simulink model "DriverInLoopGamingEngine"  (R2020b)
settings: Solver=ode3  StartTime=0.0  StopTime=inf  FixedStep=1e-3  RelTol=1e-3
StartFcn:
  | tg.load('DriverInLoopSpeedgoat');
  | tg.start;
StopFcn:
  | tg.stop;
model workspace (MAT data in the model file):
  A_mu = 10
  AxlIxx = 62.3745166667
  AxlM = 160
  B_reff = 8.386
  Cps = 2
  Cz = 5565.2246438
  CzWhlAxl = 11490.971257
  DCT_Param : object (value not decoded)
  DLC_XEnd = 236.9
  DLC_XStart = 175.9
  D_reff = 0.25826
  Downshift_Speeds = [9.5625 12.9375 16.3125 19.6875 23.0625 26.4375 29.8125 33.1875 36.5625 39.9375 43.3125 46.6875 ... (28 elements, 4x7)]
  F0z = [2886 2907]
  F0zWhlAxl = 2907
  Hmax = 0.25
  Kz = 52451.0065793
  KzWhlAxl = 138031.612078
  NCyl = 6
  Pedal_Positions = [0.1 0.4 0.5 0.9]
  Pstd = 101325
  Rair = 287
  SUS : object (value not decoded)
  Sig : Simulink.Signal (value not decoded)
  Sig1 : Simulink.Signal (value not decoded)
  Sig2 : Simulink.Signal (value not decoded)
  Sig3 : Simulink.Signal (value not decoded)
  Sig4 : Simulink.Signal (value not decoded)
  Sig5 : Simulink.Signal (value not decoded)
  Sig6 : Simulink.Signal (value not decoded)
  Sig7 : Simulink.Signal (value not decoded)
  Sig8 : Simulink.Signal (value not decoded)
  Trans : object (value not decoded)
  Tstd = 293.15
  Upshift_Speeds = [12.9375 16.3125 19.6875 33 26.4375 29.8125 33.1875 52.5 39.9375 43.3125 46.6875 77.25 ... (28 elements, 4x7)]
  VEH : object (value not decoded)
  V_o = 16.7
  V_xlow = 1
  Vd = 0.00346
  WH : Mass (value not decoded)
  Y0 = 3.2153
  a = 1.4
  alpha_max = 1.5
  alpha_min = -1.5
  b = 1.8
  c_zo = 209651
  dt3D = 0.05
  epsilon = 0.1
  f_air = [0 0 0 0 0 0 0 0 0 0 0 0 ... (256 elements, 16x16)]
  f_co = [0 0 0 0 0 0 0 0 0 0 0 0 ... (256 elements, 16x16)]
  f_co2 = [0 0 0 0 0 0 0 0 0 0 0 0 ... (256 elements, 16x16)]
  f_eff = [352.135682859 352.135682859 320.724378192 303.655312657 295.930136708 291.240087194 291.240271258 291.240312459 291.240275452 291.240198499 291.240100781 291.240018769 ... (256 elements, 16x16)]
  f_fuel = [0 0 0 0 0 0 0 0 0 0 0 0 ... (256 elements, 16x16)]
  f_hc = [0 0 0 0 0 0 0 0 0 0 0 0 ... (256 elements, 16x16)]
  f_nox = [0 0 0 0 0 0 0 0 0 0 0 0 ... (256 elements, 16x16)]
  f_pm = [0 0 0 0 0 0 0 0 0 0 0 0 ... (256 elements, 16x16)]
  f_susp_axl_bp = [1 2]
  f_susp_dz_bp = [-0.325022776267 -0.315022776267 -0.305022776267 -0.205022776267 -0.105022776267 -0.00502277626717 0.0949772237328 0.194977223733 0.204977223733 0.214977223733]
  f_susp_dzdot_bp = [-3 -0.3 -0.2 -0.1 0 0.1 0.2 0.3 3]
  f_susp_fmz = [-144070.391448 -93629.24037 -75929.1118915 -20630.5828179 -15385.48216 -10140.3815021 -4895.28084414 349.819813785 -31916.3973792 18437.6709544 -83996.1993354 -33555.0482577 ... (43920 elements, 10x9x61x2x4)]
  f_susp_geom = [0 0 0 0 0 0 0 0 0 0 0 0 ... (3660 elements, 10x61x2x3)]
  f_susp_strgdelta_bp = [-0.523598775598 -0.506145483078 -0.488692190558 -0.471238898038 -0.453785605519 -0.436332312999 -0.418879020479 -0.401425727959 -0.383972435439 -0.366519142919 -0.349065850399 -0.331612557879 ... (61 elements, 1x61)]
  f_tbrake = [0 76.8593923996 105.140482948 131.533638111 157.926793274 176.658631717 176.65727296 176.656856686 176.656879077 176.657093756 176.657404516 176.65772406 ... (256 elements, 16x16)]
  f_tbrake_n_bpt = [0 649.519052838 912.419621844 1175.32019085 1438.22075986 1701.12132886 1964.02189787 2226.92246687 2489.82303588 2752.72360489 3015.62417389 3278.5247429 ... (16 elements, 1x16)]
  f_tbrake_t_bpt = [0 34.6410161514 61.0341713143 87.4273264773 113.82048164 140.213636803 166.606791966 192.999947129 219.393102292 245.786257455 272.179412618 298.572567781 ... (16 elements, 1x16)]
  f_texh = [766.752464599 766.752464599 786.17542386 801.679939032 884.591982581 910.574397722 910.571871054 910.570774534 910.570601632 910.570821151 910.571247242 910.571639815 ... (256 elements, 16x16)]
  f_twc_eff_co = [0.17 0.25 0.45 0.99 0.99 0.99 0.99]
  f_twc_eff_hc = [0.21 0.375 0.75 0.98 0.98 0.98 0.98]
  f_twc_eff_lam = [0.909090909 0.944055944 0.979020979 1 1.013986014 1.048951049 1.083916084]
  f_twc_eff_nox = [0.98 0.98 0.98 0.97 0.05 0.02 0]
  h = 0.134
  numWheel = 4
  path : object (value not decoded)
  pio = 220000
  q_Fcx = 0
  q_Fz2 = 15.4
  q_Fzy = 0
  q_reo = 0.9974
  q_sx1 = -0.007764
  q_sx10 = 0.2824
  q_sx11 = 5.349
  q_sx12 = 0
  q_sx13 = 0
  q_sx14 = 0
  q_sx2 = 1.1915
  q_sx3 = 0.013948
  q_sx4 = 4.912
  q_sx5 = 1.02
  q_sx6 = 22.83
  q_sx7 = 0.7104
  q_sx8 = -0.023393
  q_sx9 = 0.6581
  q_sy1 = 0.00702
  q_sy2 = 0
  q_sy3 = 0.001515
  q_sy4 = 8.514e-05
  q_sy5 = 0
  q_sy6 = 0
  q_sy7 = 0.9008
  q_sy8 = -0.4089
  q_v1 = 0.0007742
  q_v2 = 0.04667
  r_Bx1 = 12.531
  r_Bx2 = 9.532
  r_Bx3 = 0
  r_By1 = 10.615
  r_By2 = 7.705
  r_By3 = 3.433e-06
  r_By4 = 0
  r_Cx1 = 1.019
  r_Cy1 = 1.0585
  r_Ex1 = -0.4487
  r_Ex2 = -0.4726
  r_Ey1 = 0.3132
  r_Ey2 = 7.63e-06
  r_Hx1 = 0.0002374
  r_Hy1 = 0.011646
  r_Hy2 = 7.63e-06
  r_Vy1 = 0.05654
  r_Vy2 = 7.63e-06
  r_Vy3 = 0
  r_Vy4 = 99.9
  r_Vy5 = 2
  r_Vy6 = 15.814
  r_o = 0.3135
  vehWidth = 2
  w = 1
  xdot_ref = 13.4112
symbols that are objects in the model workspace (value not decoded): VEH
libraries: slrealtimeutilitieslib x3, slrealtimeiplib x3, sim3dlib x2, sim3dautolib x1, dspfdesign x1, vrlib x1, simulink x1
(part 2 of 2)

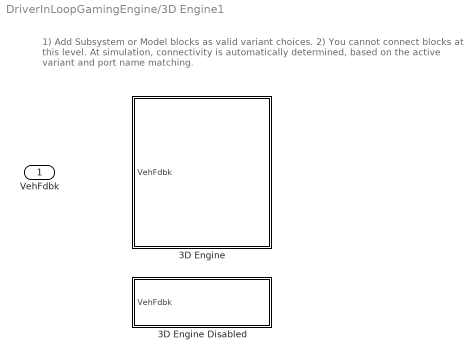
== system DriverInLoopGamingEngine/3D Engine1 ==
  note: 1) Add Subsystem or Model blocks as valid variant choices.
      | 2) You cannot connect blocks at this level. At simulation, connectivity is automatically
      | determined, based on the active variant and port name matching.
  VehFdbk : Inport
  3D Engine : Subsystem  VariantControl=1
  3D Engine Disabled : Subsystem  VariantControl=0

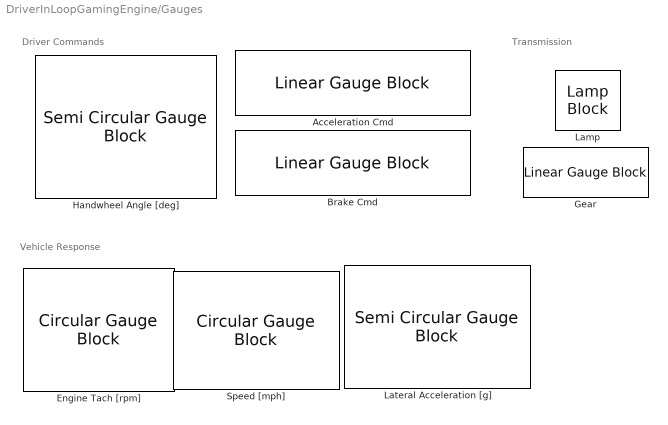
== system DriverInLoopGamingEngine/Gauges ==
  note: Vehicle Response
  note: Driver Commands
  note: Transmission
  Acceleration Cmd : LinearGaugeBlock  ScaleMax=1
  Brake Cmd : LinearGaugeBlock  ScaleMax=1
  Engine Tach [rpm] : CircularGaugeBlock  ScaleMax=8000  TickInterval=1000
  Gear : LinearGaugeBlock  ScaleMin=-1  ScaleMax=5  TickInterval=1
  Handwheel Angle [deg] : SemiCircularGaugeBlock  ScaleMin=-450  ScaleMax=450  TickInterval=90
  Lamp : LampBlock
  Lateral Acceleration [g] : SemiCircularGaugeBlock  ScaleMin=-1  ScaleMax=1  TickInterval=0.5
  Speed [mph] : CircularGaugeBlock

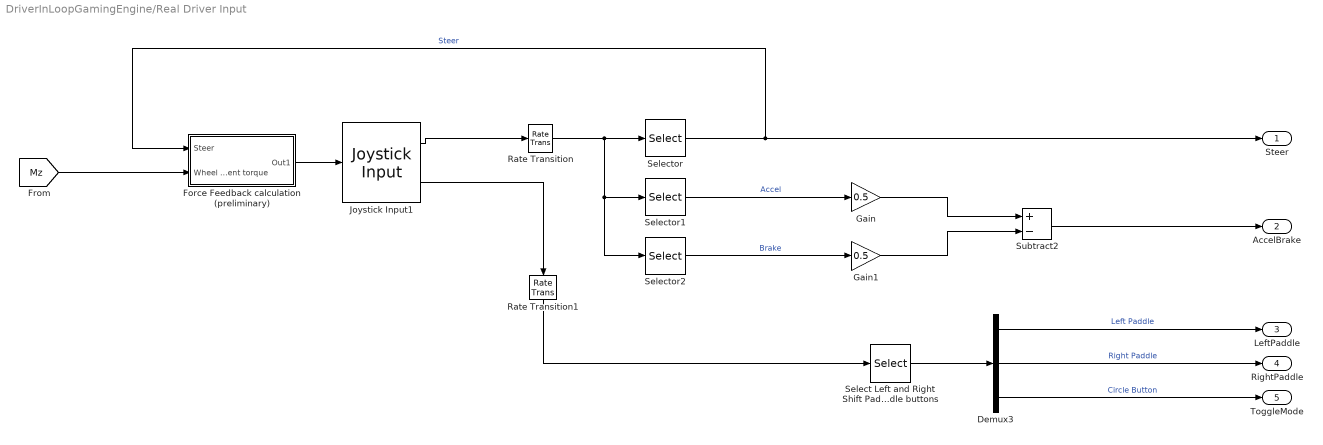
== system DriverInLoopGamingEngine/Real Driver Input ==
  Demux3 : Demux  Outputs=3
  Force Feedback calculation (preliminary) : Subsystem
  Gain : Gain  Gain=0.5
  Gain1 : Gain  Gain=0.5
  Joystick Input1 : vrlib/Joystick Input  joyid=1  adjustports=on  forcefeed=on
  Rate Transition : RateTransition  Deterministic=off
  Rate Transition1 : RateTransition  Deterministic=off
  Select Left and Right Shift Paddle buttons : Selector  InputPortWidth=25  IndexOptions=Index vector (dialog)  Indices=[6 5 3]  OutputSizes=1
  Selector : Selector  InputPortWidth=4  IndexOptions=Index vector (dialog)  Indices=1  OutputSizes=1
  Selector1 : Selector  InputPortWidth=4  IndexOptions=Index vector (dialog)  Indices=2  OutputSizes=1
  Selector2 : Selector  InputPortWidth=4  IndexOptions=Index vector (dialog)  Indices=3  OutputSizes=1
  Subtract2 : Sum  Inputs=+-
  Steer : Outport  VectorParamsAs1DForOutWhenUnconnected=off
  AccelBrake : Outport  Port=2  VectorParamsAs1DForOutWhenUnconnected=off
  LeftPaddle : Outport  Port=3  VectorParamsAs1DForOutWhenUnconnected=off
  RightPaddle : Outport  Port=4  VectorParamsAs1DForOutWhenUnconnected=off
  ToggleMode : Outport  Port=5  VectorParamsAs1DForOutWhenUnconnected=off
  wires:
  Joystick Input1/1 -> Rate Transition/1
  Rate Transition1/1 -> Select Left and Right Shift Paddle buttons/1
  Demux3/2 -> RightPaddle/1  "Right Paddle"
  Demux3/1 -> LeftPaddle/1  "Left Paddle"
  Select Left and Right Shift Paddle buttons/1 -> Demux3/1
  Rate Transition/1 -> Selector2/1, Selector1/1, Selector/1
  Joystick Input1/2 -> Rate Transition1/1
  Selector1/1 -> Gain/1  "Accel"
  Selector2/1 -> Gain1/1  "Brake"
  Gain/1 -> Subtract2/1
  Gain1/1 -> Subtract2/2
  Subtract2/1 -> AccelBrake/1
  Demux3/3 -> ToggleMode/1  "Circle Button"
  Selector/1 -> Steer/1, Force Feedback calculation (preliminary)/1(Steer)  "Steer"
  [Mz] -> Force Feedback calculation (preliminary)/2(Wheel alignment torque)
  Force Feedback calculation (preliminary)/1(Out1) -> Joystick Input1/1

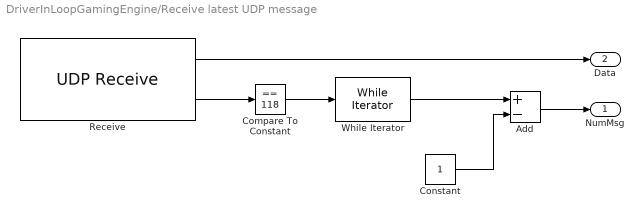
== system DriverInLoopGamingEngine/Receive latest UDP message ==
  Add : Sum  Inputs=+-
  Compare To Constant : simulink/Logic and Bit Operations/Compare To Constant  relop===  const=118  OutDataTypeStr=boolean
  Constant : Constant  OutDataTypeStr=Inherit: Inherit via back propagation  SampleTime=-1
  Receive : slrealtimeiplib/UDP Receive  useHostTargetConn=off  ipAddress=192.168.7.2  localPort=25001  rcvWidth=118  rcvFmAny=off  fmAddress=192.168.7.1  rcvMulticast=off  multicastAddress=[]  sampleTime=-1
      settings: SourceProductBaseCode=XP
  While Iterator : WhileIterator  MaxIters=10  WhileBlockType=do-while  ShowIterationPort=on
  NumMsg : Outport
  Data : Outport  Port=2
  wires:
  Receive/2 -> Compare To Constant/1
  Compare To Constant/1 -> While Iterator/1
  While Iterator/1 -> Add/1
  Constant/1 -> Add/2
  Receive/1 -> Data/1
  Add/1 -> NumMsg/1

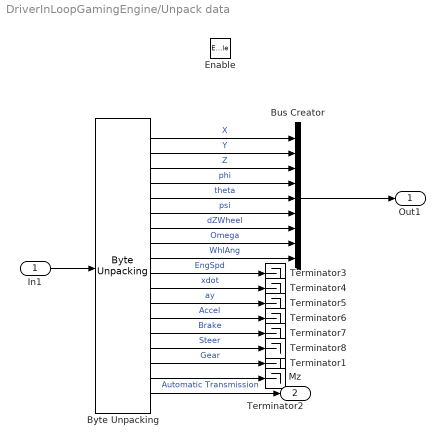
== system DriverInLoopGamingEngine/Unpack data ==
  In1 : Inport
  Enable : EnablePort
  Bus Creator : BusCreator  Inputs=9
  "Byte Unpacking " : slrealtimeutilitieslib/Byte Unpacking  MaskUnpackedDataTypes={'single','single','single','single','single','single','single','double','single','single','single','single','single','single','single','int8','int8','single'}  MaskUnpackedDataSizes={[1],[1],[1],[1],[1],[1],[4],[4],[4],[1],[1],[1],[1],[1],[1],[1],[1],[1]}  MaskAlignment=1
      settings: SourceProductBaseCode=XP
  Terminator{1..8} (8 alike) : Terminator
  Out1 : Outport
  Mz : Outport  Port=2
  wires:
  "Byte Unpacking "/8 -> Bus Creator/8  "Omega"
  "Byte Unpacking "/14 -> Terminator7/1  "Brake"
  "Byte Unpacking "/7 -> Bus Creator/7  "dZWheel"
  "Byte Unpacking "/4 -> Bus Creator/4  "phi"
  "Byte Unpacking "/15 -> Terminator8/1  "Steer"
  "Byte Unpacking "/9 -> Bus Creator/9  "WhlAng"
  "Byte Unpacking "/13 -> Terminator6/1  "Accel"
  "Byte Unpacking "/2 -> Bus Creator/2  "Y"
  "Byte Unpacking "/10 -> Terminator3/1  "EngSpd"
  In1/1 -> "Byte Unpacking "/1
  "Byte Unpacking "/3 -> Bus Creator/3  "Z"
  "Byte Unpacking "/12 -> Terminator5/1  "ay"
  "Byte Unpacking "/11 -> Terminator4/1  "xdot"
  "Byte Unpacking "/1 -> Bus Creator/1  "X"
  "Byte Unpacking "/6 -> Bus Creator/6  "psi"
  "Byte Unpacking "/5 -> Bus Creator/5  "theta"
  Bus Creator/1 -> Out1/1
  "Byte Unpacking "/16 -> Terminator1/1  "Gear"
  "Byte Unpacking "/17 -> Terminator2/1  "Automatic Transmission"
  "Byte Unpacking "/18 -> Mz/1

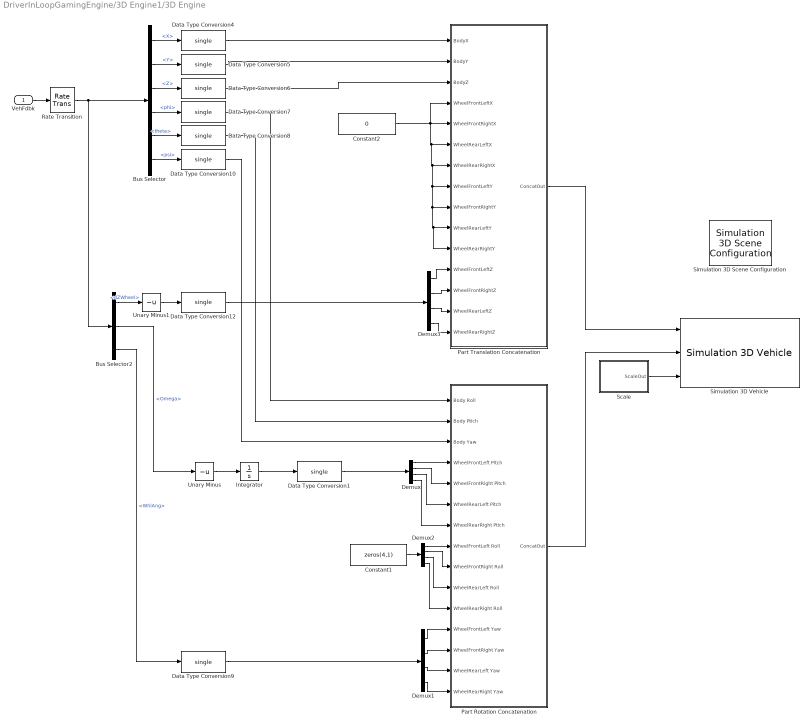
== system DriverInLoopGamingEngine/3D Engine1/3D Engine ==
  VehFdbk : Inport
  Bus Selector : BusSelector  OutputSignals=X,Y,Z,phi,theta,psi
  Bus Selector2 : BusSelector  OutputSignals=dZWheel,Omega,WhlAng
  Constant1 : Constant  Value=zeros(4,1)  OutDataTypeStr=single
  Constant2 : Constant  Value=0  OutDataTypeStr=single
  Data Type Conversion{1,4..10,12} (9 alike) : DataTypeConversion  OutDataTypeStr=single
  Demux{,1..3} (4 alike) : Demux
  Integrator : Integrator  WrapState=on  WrappedStateUpperValue=2*pi  WrappedStateLowerValue=0  ZeroCross=off
  Part Rotation Concatenation : Subsystem
  Part Translation Concatenation : Subsystem
  Rate Transition : RateTransition  Deterministic=off  OutPortSampleTime=dt3D
  Scale : Subsystem
  Simulation 3D Scene Configuration : sim3dlib/Simulation 3D Scene Configuration  Priority=0  ProjectFormat=Default Scenes  SceneDesc=Virtual Mcity  ProjectName=VehicleSimulation.exe  ScenePath=/Game/Maps/HwStrght  vehTagList={'Scene Origin';'SimulinkVehicle1'}  vehTag=SimulinkVehicle1  OpVisEn=off  Ts=dt3D  EnableWindow=on  sensorTag=MainCamera2  sensorId=2  sensorName=MainCamera2  mountLoc=Origin  offsetFlag=off  tmountOffset=[0, 0, 0]  rmountOffset=[0, 0, 0]  HorizontalResolution=1280  VerticalResolution=720  HorizontalFOV=60  mountPoint=[0 0 0]  mountOrientation=[0 0 0]  aMode=aMode  ID=2
      settings: SourceProductBaseCode=DR,UV,VE
  Simulation 3D Vehicle : sim3dautolib/Simulation 3D Vehicle  Priority=-1  PassVehMesh=Muscle car  VehColor=Red  ActorName=SimulinkVehicle1  Translation=[VEH.InitialLongPosition VEH.InitialLatPosition -VEH.InitialVertPosition; 0 0 0; 0 0 0; 0 0 0; 0 0 0]  Rotation=[VEH.InitialRollAngle VEH.InitialPitchAngle VEH.InitialYawAngle; 0 0 0; 0 0 0; 0 0 0; 0 0 0]  Scale=ones( 5, 3 )  SampleTime=dt3D  ActorType=SimulinkVehicle  ID=1  aMode=2  ActorTag=SimulinkVehicle1
      settings: SourceProductBaseCode=DR,UV,VE
  Unary Minus : UnaryMinus
  Unary Minus1 : UnaryMinus
  wires:
  Unary Minus/1 -> Integrator/1
  Bus Selector2/1 -> Unary Minus1/1  "<dZWheel>"
  Rate Transition/1 -> Bus Selector/1, Bus Selector2/1
  Scale/1(ScaleOut) -> Simulation 3D Vehicle/3
  Demux/4 -> Part Rotation Concatenation/7(WheelRearRight Ptich)
  Demux/3 -> Part Rotation Concatenation/6(WheelRearLeft Pitch)
  Demux/2 -> Part Rotation Concatenation/5(WheelFrontRight Pitch)
  Demux/1 -> Part Rotation Concatenation/4(WheelFrontLeft Pitch)
  Constant1/1 -> Demux2/1
  Bus Selector/4 -> Data Type Conversion7/1  "<phi>"
  Part Rotation Concatenation/1(ConcatOut) -> Simulation 3D Vehicle/2
  Part Translation Concatenation/1(ConcatOut) -> Simulation 3D Vehicle/1
  Data Type Conversion12/1 -> Demux3/1
  Demux3/4 -> Part Translation Concatenation/15(WheelRearRightZ)
  Demux3/3 -> Part Translation Concatenation/14(WheelRearLeftZ)
  Demux3/1 -> Part Translation Concatenation/12(WheelFrontLeftZ)
  Demux3/2 -> Part Translation Concatenation/13(WheelFrontRightZ)
  VehFdbk/1 -> Rate Transition/1
  Data Type Conversion6/1 -> Part Translation Concatenation/3(BodyZ)
  Demux1/4 -> Part Rotation Concatenation/15(WheelRearRight Yaw)
  Demux1/3 -> Part Rotation Concatenation/14(WheelRearLeft Yaw)
  Demux2/1 -> Part Rotation Concatenation/8(WheelFrontLeft Roll)
  Demux2/2 -> Part Rotation Concatenation/9(WheelFrontRight Roll)
  Demux2/3 -> Part Rotation Concatenation/10(WheelRearLeft Roll)
  Demux2/4 -> Part Rotation Concatenation/11(WheelRearRight Roll)
  Bus Selector2/3 -> Data Type Conversion9/1  "<WhlAng>"
  Bus Selector2/2 -> Unary Minus/1  "<Omega>"
  Data Type Conversion9/1 -> Demux1/1
  Demux1/1 -> Part Rotation Concatenation/12(WheelFrontLeft Yaw)
  Demux1/2 -> Part Rotation Concatenation/13(WheelFrontRight Yaw)
  Integrator/1 -> Data Type Conversion1/1
  Data Type Conversion1/1 -> Demux/1
  Data Type Conversion8/1 -> Part Rotation Concatenation/2(Body Ptich)
  Data Type Conversion5/1 -> Part Translation Concatenation/2(BodyY)
  Data Type Conversion10/1 -> Part Rotation Concatenation/3(Body Yaw)
  Constant2/1 -> Part Translation Concatenation/5(WheelFrontRightX), Part Translation Concatenation/6(WheelRearLeftX), Part Translation Concatenation/7(WheelRearRightX), Part Translation Concatenation/8(WheelFrontLeftY), Part Translation Concatenation/9(WheelFrontRightY), Part Translation Concatenation/10(WheelRearLeftY), Part Translation Concatenation/11(WheelRearRightY), Part Translation Concatenation/4(WheelFrontLeftX)
  Data Type Conversion4/1 -> Part Translation Concatenation/1(BodyX)
  Data Type Conversion7/1 -> Part Rotation Concatenation/1(Body Roll)
  Bus Selector/1 -> Data Type Conversion4/1  "<X>"
  Bus Selector/2 -> Data Type Conversion5/1  "<Y>"
  Bus Selector/3 -> Data Type Conversion6/1  "<Z>"
  Bus Selector/6 -> Data Type Conversion10/1  "<psi>"
  Bus Selector/5 -> Data Type Conversion8/1  "<theta>"
  Unary Minus1/1 -> Data Type Conversion12/1

== system DriverInLoopGamingEngine/3D Engine1/3D Engine Disabled ==
  VehFdbk : Inport
  Terminator : Terminator
  wires:
  VehFdbk/1 -> Terminator/1

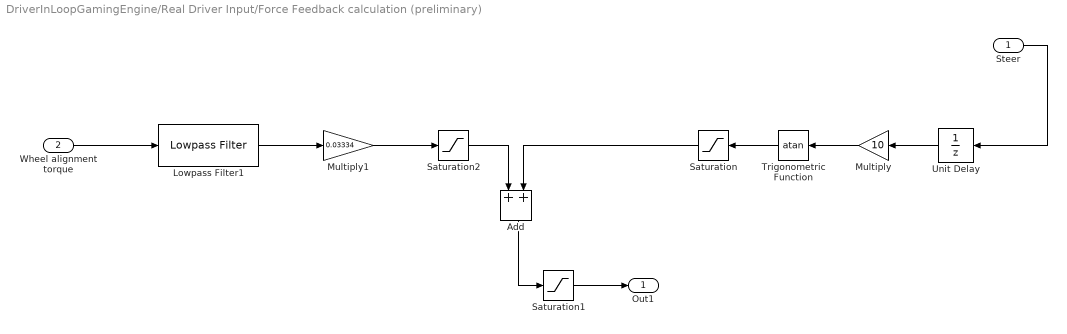
== system DriverInLoopGamingEngine/Real Driver Input/Force Feedback calculation (preliminary) ==
  Steer : Inport
  Wheel alignment torque : Inport  Port=2
  Add : Sum
  Lowpass Filter1 : dspfdesign/Lowpass Filter  FilterType=FIR  DesignForMinimumOrder=on  FilterOrder=50  PassbandFrequency=1  StopbandFrequency=40  PassbandRipple=0.1  StopbandAttenuation=80  InheritSampleRate=off  SampleRate=1000  SimulateUsing=Interpreted execution  roundingMode=Floor  coeffsDataTypeStr=fixdt(1,16)
  Multiply : Gain  Gain=10
  Multiply1 : Gain  Gain=0.03334
  Saturation : Saturate  UpperLimit=0.6  LowerLimit=-0.6
  Saturation1 : Saturate  UpperLimit=1  LowerLimit=-1
  Saturation2 : Saturate  UpperLimit=0.6  LowerLimit=-0.6
  Trigonometric Function : Trigonometry  Operator=atan  OutputSignalType=real
  Unit Delay : UnitDelay  SampleTime=-1  HasFrameUpgradeWarning=on
  Out1 : Outport
  wires:
  Multiply/1 -> Trigonometric Function/1
  Unit Delay/1 -> Multiply/1
  Saturation1/1 -> Out1/1
  Saturation/1 -> Add/2
  Multiply1/1 -> Saturation2/1
  Trigonometric Function/1 -> Saturation/1
  Add/1 -> Saturation1/1
  Lowpass Filter1/1 -> Multiply1/1
  Saturation2/1 -> Add/1
  Steer/1 -> Unit Delay/1
  Wheel alignment torque/1 -> Lowpass Filter1/1

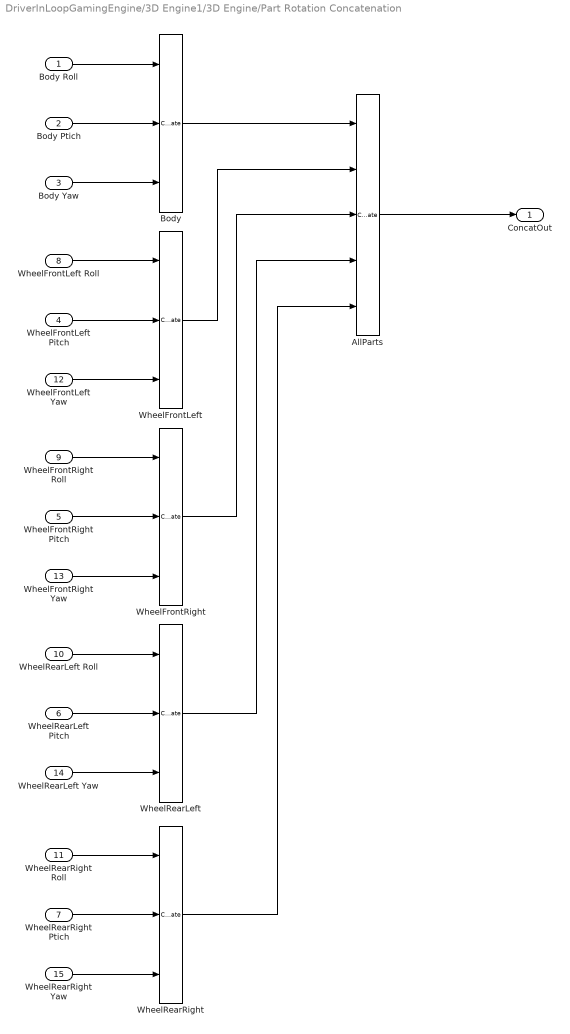
== system DriverInLoopGamingEngine/3D Engine1/3D Engine/Part Rotation Concatenation ==
  Body Roll : Inport
  Body Ptich : Inport  Port=2
  Body Yaw : Inport  Port=3
  WheelFrontLeft Pitch : Inport  Port=4
  WheelFrontRight Pitch : Inport  Port=5
  WheelRearLeft Pitch : Inport  Port=6
  WheelRearRight Ptich : Inport  Port=7
  WheelFrontLeft Roll : Inport  Port=8
  WheelFrontRight Roll : Inport  Port=9
  WheelRearLeft Roll : Inport  Port=10
  WheelRearRight Roll : Inport  Port=11
  WheelFrontLeft Yaw : Inport  Port=12
  WheelFrontRight Yaw : Inport  Port=13
  WheelRearLeft Yaw : Inport  Port=14
  WheelRearRight Yaw : Inport  Port=15
  AllParts : Concatenate  NumInputs=5  Mode=Multidimensional array
  Body : Concatenate  NumInputs=3  Mode=Multidimensional array  ConcatenateDimension=2
  WheelFrontLeft : Concatenate  NumInputs=3  Mode=Multidimensional array  ConcatenateDimension=2
  WheelFrontRight : Concatenate  NumInputs=3  Mode=Multidimensional array  ConcatenateDimension=2
  WheelRearLeft : Concatenate  NumInputs=3  Mode=Multidimensional array  ConcatenateDimension=2
  WheelRearRight : Concatenate  NumInputs=3  Mode=Multidimensional array  ConcatenateDimension=2
  ConcatOut : Outport  VectorParamsAs1DForOutWhenUnconnected=off
  wires:
  Body Yaw/1 -> Body/3
  WheelFrontLeft Yaw/1 -> WheelFrontLeft/3
  WheelFrontLeft/1 -> AllParts/2
  Body/1 -> AllParts/1
  WheelRearLeft/1 -> AllParts/4
  WheelFrontRight/1 -> AllParts/3
  WheelRearRight Yaw/1 -> WheelRearRight/3
  WheelRearLeft Yaw/1 -> WheelRearLeft/3
  AllParts/1 -> ConcatOut/1
  WheelRearRight/1 -> AllParts/5
  WheelFrontRight Yaw/1 -> WheelFrontRight/3
  Body Roll/1 -> Body/1
  Body Ptich/1 -> Body/2
  WheelFrontLeft Pitch/1 -> WheelFrontLeft/2
  WheelFrontLeft Roll/1 -> WheelFrontLeft/1
  WheelFrontRight Roll/1 -> WheelFrontRight/1
  WheelFrontRight Pitch/1 -> WheelFrontRight/2
  WheelRearLeft Roll/1 -> WheelRearLeft/1
  WheelRearLeft Pitch/1 -> WheelRearLeft/2
  WheelRearRight Roll/1 -> WheelRearRight/1
  WheelRearRight Ptich/1 -> WheelRearRight/2

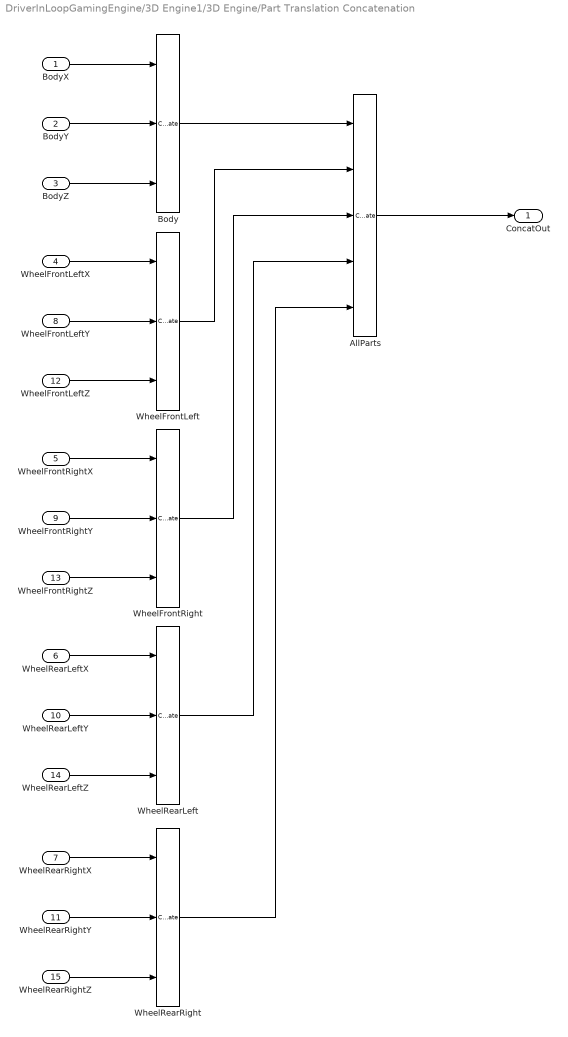
== system DriverInLoopGamingEngine/3D Engine1/3D Engine/Part Translation Concatenation ==
  BodyX : Inport
  BodyY : Inport  Port=2
  BodyZ : Inport  Port=3
  WheelFrontLeftX : Inport  Port=4
  WheelFrontRightX : Inport  Port=5
  WheelRearLeftX : Inport  Port=6
  WheelRearRightX : Inport  Port=7
  WheelFrontLeftY : Inport  Port=8
  WheelFrontRightY : Inport  Port=9
  WheelRearLeftY : Inport  Port=10
  WheelRearRightY : Inport  Port=11
  WheelFrontLeftZ : Inport  Port=12
  WheelFrontRightZ : Inport  Port=13
  WheelRearLeftZ : Inport  Port=14
  WheelRearRightZ : Inport  Port=15
  AllParts : Concatenate  NumInputs=5  Mode=Multidimensional array
  Body : Concatenate  NumInputs=3  Mode=Multidimensional array  ConcatenateDimension=2
  WheelFrontLeft : Concatenate  NumInputs=3  Mode=Multidimensional array  ConcatenateDimension=2
  WheelFrontRight : Concatenate  NumInputs=3  Mode=Multidimensional array  ConcatenateDimension=2
  WheelRearLeft : Concatenate  NumInputs=3  Mode=Multidimensional array  ConcatenateDimension=2
  WheelRearRight : Concatenate  NumInputs=3  Mode=Multidimensional array  ConcatenateDimension=2
  ConcatOut : Outport  VectorParamsAs1DForOutWhenUnconnected=off
  wires:
  BodyX/1 -> Body/1
  BodyZ/1 -> Body/3
  WheelFrontLeftX/1 -> WheelFrontLeft/1
  WheelFrontLeftZ/1 -> WheelFrontLeft/3
  WheelFrontLeftY/1 -> WheelFrontLeft/2
  BodyY/1 -> Body/2
  WheelFrontLeft/1 -> AllParts/2
  WheelRearRightX/1 -> WheelRearRight/1
  Body/1 -> AllParts/1
  WheelRearLeft/1 -> AllParts/4
  WheelFrontRight/1 -> AllParts/3
  WheelRearRightZ/1 -> WheelRearRight/3
  WheelFrontRightY/1 -> WheelFrontRight/2
  WheelFrontRightX/1 -> WheelFrontRight/1
  WheelRearRightY/1 -> WheelRearRight/2
  WheelRearLeftZ/1 -> WheelRearLeft/3
  AllParts/1 -> ConcatOut/1
  WheelRearLeftY/1 -> WheelRearLeft/2
  WheelRearRight/1 -> AllParts/5
  WheelRearLeftX/1 -> WheelRearLeft/1
  WheelFrontRightZ/1 -> WheelFrontRight/3

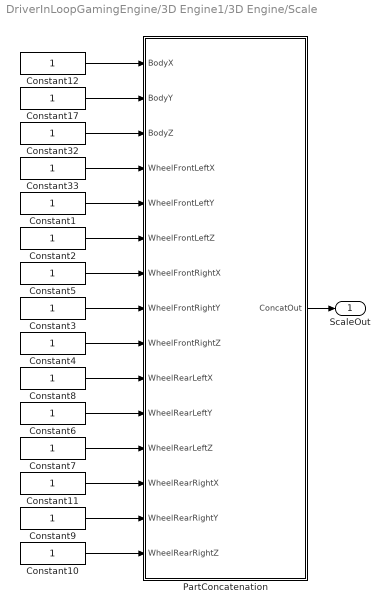
== system DriverInLoopGamingEngine/3D Engine1/3D Engine/Scale ==
  Constant{1..12,17,32..33} (15 alike) : Constant  OutDataTypeStr=single
  PartConcatenation : Subsystem
  ScaleOut : Outport  VectorParamsAs1DForOutWhenUnconnected=off
  wires:
  Constant10/1 -> PartConcatenation/15(WheelRearRightZ)
  Constant9/1 -> PartConcatenation/14(WheelRearRightY)
  Constant11/1 -> PartConcatenation/13(WheelRearRightX)
  Constant7/1 -> PartConcatenation/12(WheelRearLeftZ)
  Constant6/1 -> PartConcatenation/11(WheelRearLeftY)
  Constant8/1 -> PartConcatenation/10(WheelRearLeftX)
  Constant4/1 -> PartConcatenation/9(WheelFrontRightZ)
  Constant3/1 -> PartConcatenation/8(WheelFrontRightY)
  Constant5/1 -> PartConcatenation/7(WheelFrontRightX)
  Constant2/1 -> PartConcatenation/6(WheelFrontLeftZ)
  Constant1/1 -> PartConcatenation/5(WheelFrontLeftY)
  Constant33/1 -> PartConcatenation/4(WheelFrontLeftX)
  Constant32/1 -> PartConcatenation/3(BodyZ)
  Constant17/1 -> PartConcatenation/2(BodyY)
  Constant12/1 -> PartConcatenation/1(BodyX)
  PartConcatenation/1(ConcatOut) -> ScaleOut/1

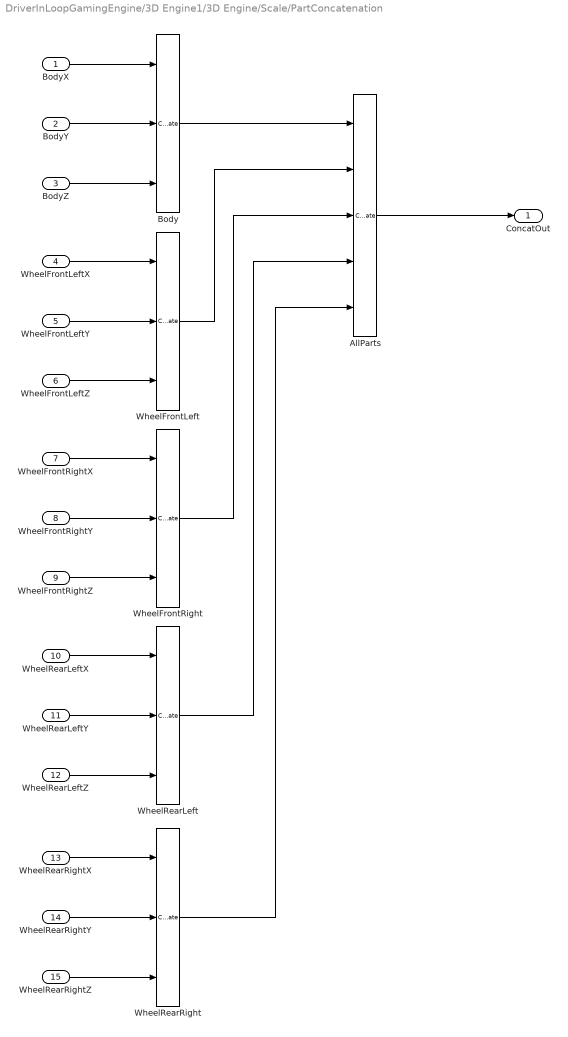
== system DriverInLoopGamingEngine/3D Engine1/3D Engine/Scale/PartConcatenation ==
  BodyX : Inport
  BodyY : Inport  Port=2
  BodyZ : Inport  Port=3
  WheelFrontLeftX : Inport  Port=4
  WheelFrontLeftY : Inport  Port=5
  WheelFrontLeftZ : Inport  Port=6
  WheelFrontRightX : Inport  Port=7
  WheelFrontRightY : Inport  Port=8
  WheelFrontRightZ : Inport  Port=9
  WheelRearLeftX : Inport  Port=10
  WheelRearLeftY : Inport  Port=11
  WheelRearLeftZ : Inport  Port=12
  WheelRearRightX : Inport  Port=13
  WheelRearRightY : Inport  Port=14
  WheelRearRightZ : Inport  Port=15
  AllParts : Concatenate  NumInputs=5  Mode=Multidimensional array
  Body : Concatenate  NumInputs=3  Mode=Multidimensional array  ConcatenateDimension=2
  WheelFrontLeft : Concatenate  NumInputs=3  Mode=Multidimensional array  ConcatenateDimension=2
  WheelFrontRight : Concatenate  NumInputs=3  Mode=Multidimensional array  ConcatenateDimension=2
  WheelRearLeft : Concatenate  NumInputs=3  Mode=Multidimensional array  ConcatenateDimension=2
  WheelRearRight : Concatenate  NumInputs=3  Mode=Multidimensional array  ConcatenateDimension=2
  ConcatOut : Outport  VectorParamsAs1DForOutWhenUnconnected=off
  wires:
  BodyX/1 -> Body/1
  BodyZ/1 -> Body/3
  WheelFrontLeftX/1 -> WheelFrontLeft/1
  WheelFrontLeftZ/1 -> WheelFrontLeft/3
  WheelFrontLeftY/1 -> WheelFrontLeft/2
  BodyY/1 -> Body/2
  WheelFrontLeft/1 -> AllParts/2
  WheelRearRightX/1 -> WheelRearRight/1
  Body/1 -> AllParts/1
  WheelRearLeft/1 -> AllParts/4
  WheelFrontRight/1 -> AllParts/3
  WheelRearRightZ/1 -> WheelRearRight/3
  WheelFrontRightY/1 -> WheelFrontRight/2
  WheelFrontRightX/1 -> WheelFrontRight/1
  WheelRearRightY/1 -> WheelRearRight/2
  WheelRearLeftZ/1 -> WheelRearLeft/3
  AllParts/1 -> ConcatOut/1
  WheelRearLeftY/1 -> WheelRearLeft/2
  WheelRearRight/1 -> AllParts/5
  WheelRearLeftX/1 -> WheelRearLeft/1
  WheelFrontRightZ/1 -> WheelFrontRight/3
